simulink model "Copy_of_Ball_Estimation"  (Simulink 8.1)
settings: Solver=ode4  StartTime=0.0  StopTime=inf  FixedStep=sample_time  RelTol=1e-3
InitFcn:
  | sample_time=0.005;%0.004;%0.0025;%0.02;
  | sample_time_Vicon = 0.005;
  | DeltaT = 0.02;
  | g = 9.81;
  | H0 = g%0.3165;
  | Kl = 1;
  | 
  | Omega_r = 1.6;%for Horizontal reference
  | Zeta_r = 0.7; %for Horizontal reference
  | Omega = 1.8;%for Horizontal Control
  | Zeta = 0.5;    %for Horizontal Control
  | 
  | Omega_h_r = 2.2; %for vertical reference
  | Zeta_h_r = 0.8;  %for vertical reference
  | Omega_h = 2.3;    %for vertical control
  | Zeta_h = 0.8;         %for vertical control
  | PI=pi;
  | 
  | Mass = 1;
  | Acc_Max = 4;
  | Acc_Max_h = 4;
  | 
  | Max_RP = 60;
  | 
  | % for NN
  | n = 5;
  | r = 3;
  | n2 = 5;
  | NN_ST = 0.02;
  | 
  | GAMA_V = 6;
  | gama_V_e = 0.01;
  | 
  | GAMA_W = GAMA_V;
  | gama_W_e =0.01;
  | 
  | % deadzone
  | NN_Deadzone_Z = 0;
  | 
  | % inputs nomalizaton parameters
  | NN_Z_y_min = -3;
  | NN_Z_y_max = 0.5;
  | 
  | NN_Z_v_max = 8;
  | NN_Z_v_min = -NN_Z_v_max;
  | 
  | % alpha = 0.034;
  | alpha = 1;
  | % c_f = 0.0015;
  | c_f = 0.001;
  | c_y_tilt = 1*0.5;
libraries: simulink x2
settings Model: Creator=ttcl3  LastModifiedBy=Vicon
settings SolverCC: MaxConsecutiveMinStep=auto
settings DebuggingCC: MultiTaskRateTransMsg=warning
settings SFSimCC: SimParseCustomCode=off

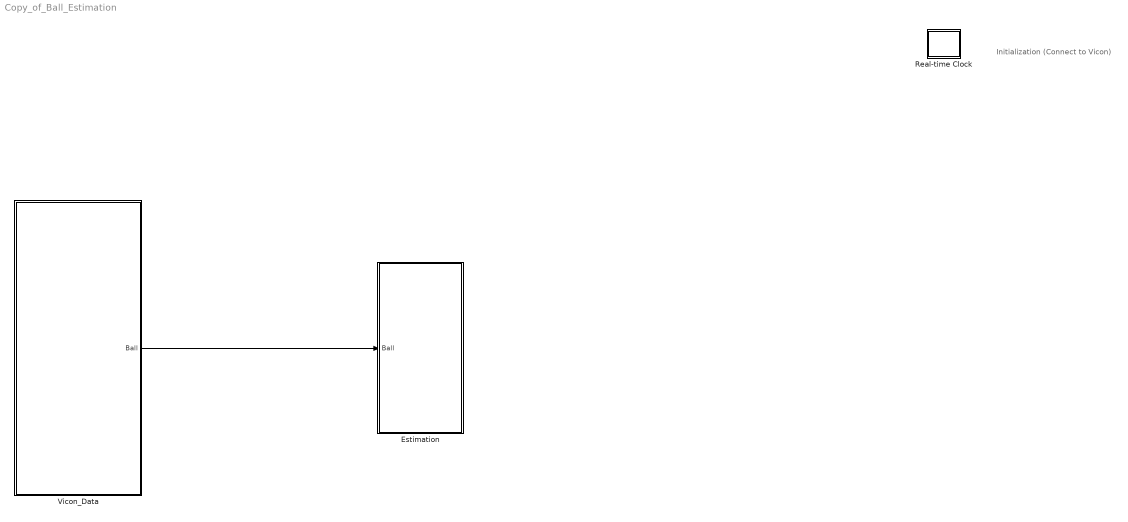
== system Copy_of_Ball_Estimation ==
  note: Initialization
      | (Connect to Vicon)
  Estimation : Subsystem
  Real-time Clock : Subsystem  mask(Real-time Clock){sample_time=0.02, tolerance=1}
      mask prompts: sample_time "Synchronize with real-time every n seconds:"; tolerance "Real-time warning tolerance (seconds):"
      mask help: Real-time Synchronization Block
      mask Help: This block synchronizes simulation time with the PC real-time clock or UNIX system clock. The first dialog entry is the period at which the clock is checked to insure real-time synchronization. The second dialog entry is the number of seconds that the simulation time must be within real-time before a warning is printed.
      mask Display: plot(0,0,100,100,[40,60,60,54,54,64,69,76,82,77,81,83,83,81,78,74,70,64,57,49,41,35,32,30,30,31,34,40,47,47,40,40],[90,90,85,85,80,79,76,87,80,70,64,57,49,41,33,28,24,22,21,23,25,31,37,46,56,65,73,78,80,85,85,90],[69,53,53],[64,50,73])
  Vicon_Data : Subsystem
  wires:
  Vicon_Data/1(Ball) -> Estimation/1(Ball)

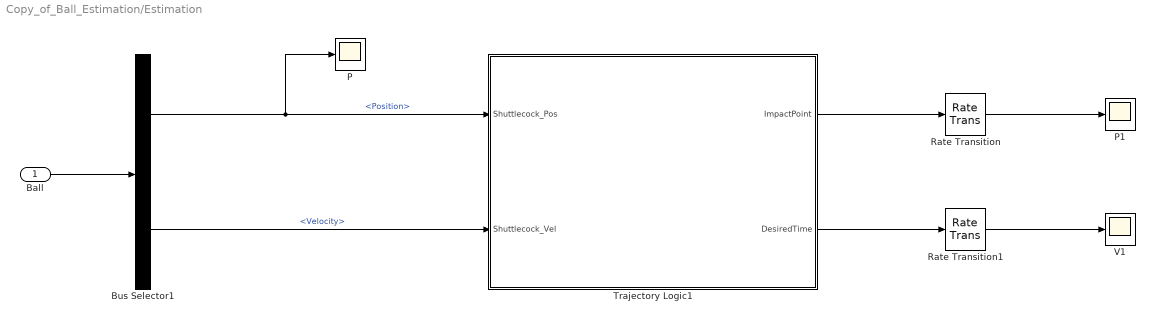
== system Copy_of_Ball_Estimation/Estimation ==
  Ball : Inport
  Bus Selector1 : BusSelector  OutputSignals=Position,Velocity
  P : Scope
      settings: MaxDataPoints=50000
  P1 : Scope
      settings: SaveName=ScopeData4  MaxDataPoints=50000
  Rate Transition : RateTransition  OutPortSampleTime=0.02
  Rate Transition1 : RateTransition  OutPortSampleTime=0.02
  Trajectory Logic1 : Subsystem
  V1 : Scope
      settings: SaveName=ScopeData5
  wires:
  Ball/1 -> Bus Selector1/1
  Bus Selector1/1 -> P/1, Trajectory Logic1/1(Shuttlecock_Pos)  "<Position>"
  Bus Selector1/2 -> Trajectory Logic1/2(Shuttlecock_Vel)  "<Velocity>"
  Trajectory Logic1/1("ImpactPoint ") -> Rate Transition/1
  Trajectory Logic1/2(DesiredTime) -> Rate Transition1/1
  Rate Transition/1 -> P1/1
  Rate Transition1/1 -> V1/1

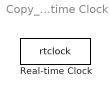
== system Copy_of_Ball_Estimation/Real-time Clock ==
  Real-time Clock : S-Function  FunctionName=rtclock  Parameters=sample_time, tolerance  EnableBusSupport=off

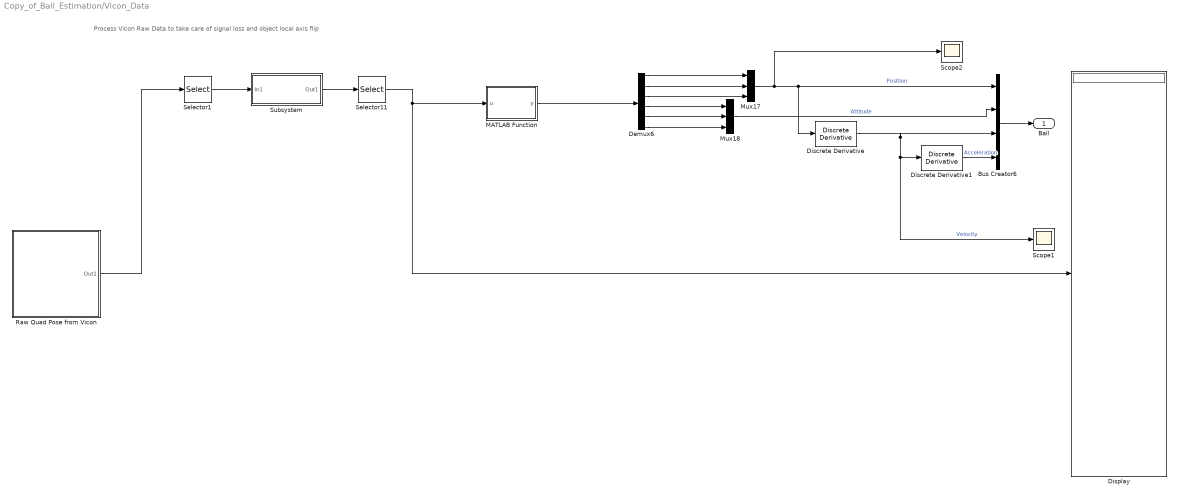
== system Copy_of_Ball_Estimation/Vicon_Data ==
  note: Process Vicon Raw Data to take care of signal loss and object local axis flip
  Bus Creator6 : BusCreator
  Demux6 : Demux  Outputs=6
  Discrete Derivative : simulink/Discrete/Discrete Derivative  gainval=1.0  ICPrevScaledInput=0.0  InputProcessing=Inherited  OutMin=[]  OutMax=[]  OutDataType=fixdt(1, 16)  OutScaling=2^-10  DoSatur=off
  Discrete Derivative1 : simulink/Discrete/Discrete Derivative  gainval=1.0  ICPrevScaledInput=0.0  InputProcessing=Inherited  OutMin=[]  OutMax=[]  OutDataType=fixdt(1, 16)  OutScaling=2^-10  DoSatur=off
  Display : Display
  MATLAB Function : MATLAB Function  TreatAsAtomicUnit=on
  Mux17 : Mux  Inputs=3
  Mux18 : Mux  Inputs=3
  Raw Quad Pose from Vicon : Subsystem
  Scope1 : Scope
      settings: YMin=-300  YMax=50
  Scope2 : Scope
      settings: YMin=-3  YMax=4.5
  Selector1 : Selector  InputPortWidth=30  IndexOptions=Index vector (dialog)  Indices=[1 2 3 ]  OutputSizes=1
  Selector11 : Selector  InputPortWidth=6  IndexOptions=Index vector (dialog)  Indices=[1 2 3 ]  OutputSizes=1
  Subsystem : Subsystem
  Ball : Outport
  wires:
  Demux6/6 -> Mux18/3
  Mux17/1 -> Scope2/1, Bus Creator6/1, Discrete Derivative/1  "Position"
  Bus Creator6/1 -> Ball/1
  Raw Quad Pose from Vicon/1(Out1) -> Selector1/1
  Selector1/1 -> Subsystem/1(In1)
  MATLAB Function/1(y) -> Demux6/1
  Subsystem/1(Out1) -> Selector11/1
  Selector11/1 -> Display/1, MATLAB Function/1(u)
  Demux6/5 -> Mux18/2
  Demux6/4 -> Mux18/1
  Mux18/1 -> Bus Creator6/2  "Attitude"
  Demux6/1 -> Mux17/1
  Demux6/2 -> Mux17/2
  Demux6/3 -> Mux17/3
  Discrete Derivative/1 -> Discrete Derivative1/1, Scope1/1, Bus Creator6/3  "Velocity"
  Discrete Derivative1/1 -> Bus Creator6/4  "Acceleration"

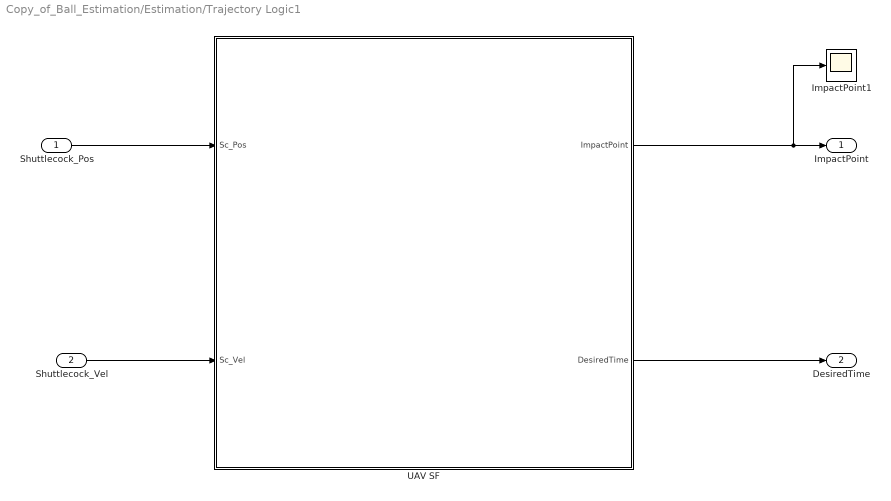
== system Copy_of_Ball_Estimation/Estimation/Trajectory Logic1 ==
  Shuttlecock_Pos : Inport
  Shuttlecock_Vel : Inport  Port=2
  ImpactPoint1 : Scope
      settings: YMin=-4  YMax=4  SaveName=ScopeData2  MaxDataPoints=50000
  UAV SF : Stateflow chart  TreatAsAtomicUnit=on
  "ImpactPoint " : Outport
  DesiredTime : Outport  Port=2
  wires:
  Shuttlecock_Pos/1 -> UAV SF/1(Sc_Pos)
  Shuttlecock_Vel/1 -> UAV SF/2(Sc_Vel)
  UAV SF/1(ImpactPoint) -> "ImpactPoint "/1, ImpactPoint1/1
  UAV SF/2(DesiredTime) -> DesiredTime/1

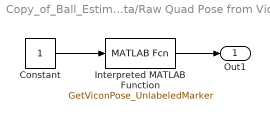
== system Copy_of_Ball_Estimation/Vicon_Data/Raw Quad Pose from Vicon ==
  Constant : Constant
  Interpreted MATLAB Function : MATLABFcn  MATLABFcn=GetViconPose_UnlabeledMarker  SampleTime=0.005
  Out1 : Outport
  wires:
  Constant/1 -> Interpreted MATLAB Function/1
  Interpreted MATLAB Function/1 -> Out1/1

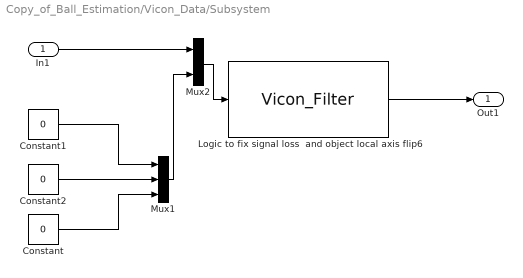
== system Copy_of_Ball_Estimation/Vicon_Data/Subsystem ==
  In1 : Inport
  Constant : Constant  Value=0
  Constant1 : Constant  Value=0
  Constant2 : Constant  Value=0
  Logic to fix signal loss  and object local axis flip6 : M-S-Function  FunctionName=Vicon_Filter
  Mux1 : Mux  Inputs=3
  Mux2 : Mux  Inputs=2
  Out1 : Outport
  wires:
  Constant1/1 -> Mux1/1
  Constant2/1 -> Mux1/2
  Mux1/1 -> Mux2/2
  Mux2/1 -> Logic to fix signal loss  and object local axis flip6/1
  Constant/1 -> Mux1/3
  In1/1 -> Mux2/1
  Logic to fix signal loss  and object local axis flip6/1 -> Out1/1

== matlab function Vicon_Data/MATLAB Function ==
  data: u input double; y output double
function y = fcn(u)
%#codegen
y = zeros(6,1);
y(1) = u(1)/1000;
y(2) = -u(2)/1000;
y(3) = -u(3)/1000;
y(4) = 0;
y(5) = 0;
y(6) = 0;
end

== stateflow chart Estimation/Trajectory Logic1/UAV SF ==
  state Airborne
    state Standby
    state Calculation
      en:
      [Pe,T]=TrajEst(x,y,z,zd,Peo[0],Peo[1],To);
      x[0] = x[1];x[1] = x[2];x[2] = x[3];x[3] = x[4];
      y[0] = y[1];y[1] = y[2];y[2] = y[3];y[3] = y[4];
      z[0] = z[1];z[1] = z[2];z[2] = z[3];z[3] = z[4];
    state Getdata
      en:
      x[i] = Sc_Pos[0];
      y[i] = Sc_Pos[1];
      z[i] = Sc_Pos[2];
    state Output1
      en:
      ImpactPoint = Pe;
      DesiredTime = T;
    state daq
      en:
      i=i+1;
    (default) -> Standby : {i=-1;Peo=0;To=0;}
    Standby -> (junction 17) : [(abs(Sc_Pos[0]) <= 4.5)&(abs(Sc_Pos[1])<=4.5)&(abs(Sc_Pos[2])<=4)]
    (junction 17) -> daq [order 1] : [(Sc_Vel[2] < -1)&(Sc_Vel[2] > -6)&(Sc_Pos[2] <-0.5)]
    (junction 17) -> Standby [order 2]
    Getdata -> daq
    daq -> Getdata [order 1] : [i==0]
    (junction 18) -> Getdata [order 1] : [(x[i-1]~=Sc_Pos[0])||(y[i-1]~=Sc_Pos[1])||(z[i-1]~=Sc_Pos[2])]
    Output1 -> daq : {i=i-2;}
    daq -> (junction 18) [order 3] : [(i>0)&(i<5)]
    (junction 18) -> daq [order 2] : {i=i-1;}
    daq -> Calculation [order 2] : [i==5]
    Calculation -> Output1 : {Peo=Pe;To=T;}
  data: xi function_input double size=5; yi function_input double size=5; zi function_input double size=5; Pe function_output double size=3; T function_output double size=1; zd function_input double size=1; t0 constant double size=5 =[0 0.02 0.04 0.06 0.08]; xo function_input double; yo function_input double; To function_input double; ImpactPoint output double size=3; DesiredTime output double size=1; Sc_Pos input double size=3; Sc_Vel input double size=3; DeltaT parameter double size=1; T local double size=1; zd local double size=1 =-0.5; Pe local double size=3; i local double; x local double size=5 =[0 0 0 0 0]; y local double size=5 =[0 0 0 0 0]; z local double size=5 =[0 0 0 0 0]; Peo local double size=3; To local double size=1
  function [Pe,T]=TrajEst(xi,yi,zi,zd,xo,yo,To):
    | function [Pe,T]=TrajEst(xi,yi,zi,zd,xo,yo,To)
    | 
    | p=polyfit(t0,zi,2)';
    | a=p(1);
    | b=p(2);
    | c=p(3);
    | 
    | 
    | xe=0;
    | ye=0;
    | T=0;
    | if((To>0)&&(To<1.2))
    |     xe = xo;
    |     ye = yo;
    |     T = To;
    | end;
    | if(a > 3)
    |     if(b^2 - 4*a*(c-zd) >= 0)
    |         T=(-b+sqrt(b^2 - 4*a*(c-zd)))/(2*a);
    |         xe=polyval(polyfit(t0,xi,1),T);
    |         ye=polyval(polyfit(t0,yi,1),T);
    |     end;
    | 
    |     if((To>0)&&(To<1.2))
    |         if((T>1.2)||(abs(xe)>4)||(abs(ye)>4))
    |             T = To;
    |             xe = xo;
    |             ye = yo;
    |         else
    |             T = 0.7*T + 0.3*(To-0.005);
    |             xe = 0.7*xo + 0.3*xe;
    |             ye = 0.7*yo + 0.3*ye;
    |         end
    |     else
    |        if((T>1.2)||(abs(xe)>4)||(abs(ye)>4)) 
    |            xe=0;
    |            ye=0;
    |            T=0;
    |        end;
    |     end;
    | end
    | 
    | Pe=[xe ye zd]';
